simulink model "mecanum_chassis_force_feedback"  (R2024b)
settings: Solver=VariableStepAuto  StartTime=0.0  StopTime=10.0  RelTol=1e-3
undefined symbols (not defined in the file): DiscIntNeverNeededParam, Ke, Kt, mu_wheel, n, Ra, Rw, Ts, Vmax
libraries: motor_jgb37 x1, simulink x1
settings Model: DataDictionary=mecanum_params.sldd  Creator=Austinchao  LastModifiedBy=Austinchao

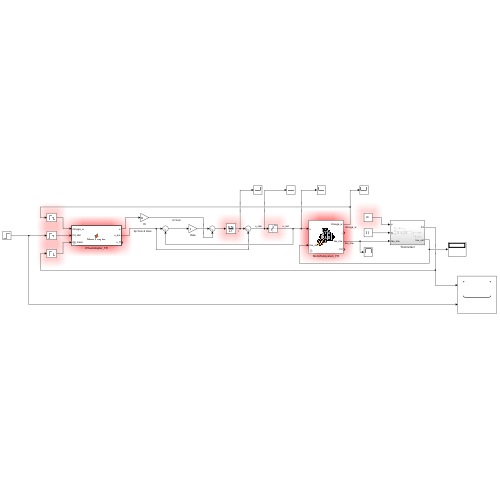
[thumbnail: Simulink's stored preview of the top-level diagram]
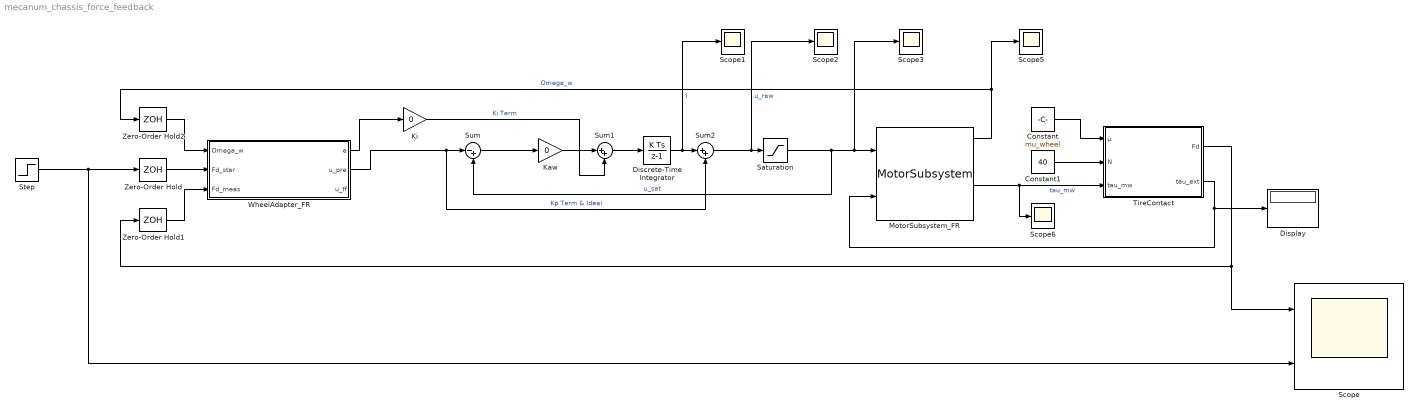
== system mecanum_chassis_force_feedback ==
  Constant : Constant  Value=mu_wheel
  Constant1 : Constant  Value=40
  Discrete-Time Integrator : DiscreteIntegrator  SampleTime=Ts  ICPrevOutput=DiscIntNeverNeededParam  ICPrevScaledInput=DiscIntNeverNeededParam
  Display : Display
  Kaw : Gain  Gain=0
  Ki : Gain  Gain=0
  MotorSubsystem_FR : motor_jgb37/MotorSubsystem  Ra=Ra  Kt=Kt  Ke=Ke  n=n  Rw=Rw  Jm=1*10^-5  Jw=1*10^-4  Bm=3.95*10^-7  tau_c=0  dz=0  Ts=Ts  Bw=0
      settings: SourceProductName=My Library
  Saturation : Saturate  UpperLimit=Vmax  LowerLimit=0
  Scope : Scope  NumInputPorts=2
  Scope{1..3,5..6} (5 alike) : Scope
  Step : Step  Time=0.2  After=12  SampleTime=0
  Sum : Sum  Inputs=|-+
  Sum1 : Sum  Inputs=|++
  Sum2 : Sum  Inputs=|++
  TireContact : Subsystem
  WheelAdapter_FR : MATLAB Function  TreatAsAtomicUnit=on  mask{Rw=Rw, n=n, Ra=Ra, Kt=Kt, Ke=Ke, Ts=Ts, Kp=0}
      mask prompts: Rw "Rw: Wheel radius (m)"; n "n: Gear ratio"; Ra "Ra: Armature resistance (Ohm)"; Kt "Kt: Torque constant (Nm/A)"; Ke "Ke: Back-EMF constant (V/(rad/s))"
  Zero-Order Hold : ZeroOrderHold  SampleTime=Ts
  Zero-Order Hold1 : ZeroOrderHold  SampleTime=Ts
  Zero-Order Hold2 : ZeroOrderHold  SampleTime=Ts
  wires:
  WheelAdapter_FR/1(e) -> Ki/1
  Discrete-Time Integrator/1 -> Scope1/1, Sum2/1  "I"
  Sum1/1 -> Discrete-Time Integrator/1
  Sum/1 -> Kaw/1
  Zero-Order Hold2/1 -> WheelAdapter_FR/1(Omega_w)
  Step/1 -> Scope/2, Zero-Order Hold/1
  Zero-Order Hold1/1 -> WheelAdapter_FR/3(Fd_meas)
  Constant1/1 -> TireContact/2(N)
  TireContact/1(Fd) -> Zero-Order Hold1/1, Scope/1
  Zero-Order Hold/1 -> WheelAdapter_FR/2(Fd_star)
  TireContact/2(tau_ext) -> Display/1, MotorSubsystem_FR/2
  MotorSubsystem_FR/3 -> Scope6/1, TireContact/3(tau_mw)  "tau_mw"
  Sum2/1 -> Scope2/1, Saturation/1  "u_raw"
  Constant/1 -> TireContact/1(μ)
  Saturation/1 -> Scope3/1, MotorSubsystem_FR/1, Sum/2  "u_sat"
  Kaw/1 -> Sum1/1
  WheelAdapter_FR/2(u_pre) -> Sum2/2, Sum/1  "Kp Term & Ideal"
  Ki/1 -> Sum1/2  "Ki Term"
  MotorSubsystem_FR/1 -> Scope5/1, Zero-Order Hold2/1  "Omega_w"

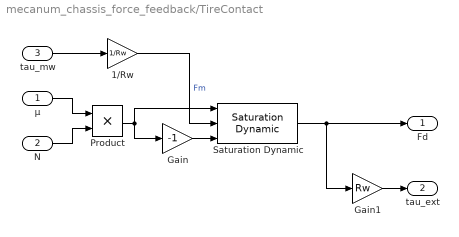
== system mecanum_chassis_force_feedback/TireContact ==
  μ : Inport
  N : Inport  Port=2
  tau_mw : Inport  Port=3
  1/Rw : Gain  Gain=1/Rw
  Gain : Gain  Gain=-1
  Gain1 : Gain  Gain=Rw
  Product : Product
  Saturation Dynamic : simulink/Discontinuities/Saturation Dynamic  OutMin=[]  OutMax=[]  OutDataTypeStr=Inherit: Same as second input  OutDataType=fixdt(1, 16)  OutScaling=2^-10  DoSatur=off
  Fd : Outport
  tau_ext : Outport  Port=2
  wires:
  tau_mw/1 -> 1/Rw/1
  μ/1 -> Product/1
  N/1 -> Product/2
  Product/1 -> Gain/1, Saturation Dynamic/1
  Gain/1 -> Saturation Dynamic/3
  1/Rw/1 -> Saturation Dynamic/2  "Fm"
  Saturation Dynamic/1 -> Gain1/1, Fd/1
  Gain1/1 -> tau_ext/1

== matlab function mecanum_chassis_force_feedback/WheelAdapter_FR ==
  data: e output; Omega_w input; Fd_star input; Fd_meas input; Rw parameter; n parameter; Ra parameter; Kt parameter; Ke parameter; Kp parameter; u_pre output; u_ff output
function [e , u_pre , u_ff] = WheelAdapter(Omega_w,Fd_star, Fd_meas, Rw, n, Ra, Kt, Ke, Kp)
%persistent I; if isempty(I), I = 0; end
% Fd_star : 期望輪力 (來自 ForceMixer)
% Fd_meas : 實際輸出輪力 (來自 MotorSubsystem)
% Omega_w : 輪速 (來自 MotorSubsystem)

% Mask 參數（之後會在 Mask 裡設定）
% Rw  : 輪半徑 [m]
% n   : 減速比
% Ra  : 電阻 [Ohm]
% Kt  : 轉矩常數 [Nm/A]
% Ke  : 反電動勢常數 [V/(rad/s)]

% 期望輪扭矩
tau_w_star = Rw * Fd_star;

% 前饋電壓
u_ff = (Ra/(Kt*n)) * tau_w_star + (Ke*n) * Omega_w;

% 誤差與比例動作
e     = Fd_star - Fd_meas;
u_pre = u_ff ;

end
